simulink model "verify_House_OneNodeModel_mdl"  (R2016b)
settings: Solver=ode45  StartTime=0.0  StopTime=2*24*3600  MaxStep=100  RelTol=1e-3  EnableMultiTasking=on
libraries: carnot x5
settings Model: Creator=drhf  LastModifiedBy=drhf
settings DataIOCC: SaveFormat=Array  SignalLoggingSaveFormat=ModelDataLogs
settings OptimizationCC: ExpressionDepthLimit=2147483647  LifeSpan=inf
settings DebuggingCC: UnderspecifiedInitializationDetection=Classic  MergeDetectMultiDrivingBlocksExec=none  SolverPrmCheckMsg=warning  FcnCallInpInsideContextMsg=warning  StateNameClashWarn=warning  SFUnexpectedBacktrackingDiag=warning  SFNoUnconditionalDefaultTransitionDiag=warning  SFExecutionAtInitializationDiag=none
settings HardwareCC: ProdBitPerPointer=32  ProdBitPerSizeT=32  ProdBitPerPtrDiffT=32  ProdLargestAtomicFloat=None  ProdIntDivRoundTo=Undefined  ProdEndianess=Unspecified  ProdWordSize=32  ProdHWDeviceType=32-bit Generic
settings ModelReferenceCC: PropagateSignalLabelsOutOfModel=off
settings GRTTargetCC: TargetLangStandard=C89/C90 (ANSI)  GeneratePreprocessorConditionals=Disable all  CombineOutputUpdateFcns=off  GRTInterface=on
settings ConfigComp: CovMetricSettings=dw  CovHtmlReporting=on  CovSaveCumulativeToWorkspaceVar=on  CovSaveSingleToWorkspaceVar=on  CovExternalEMLEnable=off

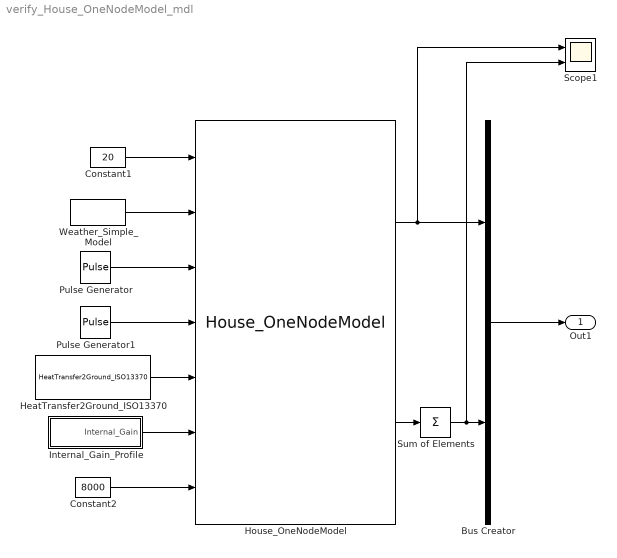
== system verify_House_OneNodeModel_mdl ==
  Bus Creator : BusCreator  Inputs=2
  Constant1 : Constant  Value=20
  Constant2 : Constant  Value=8000
  HeatTransfer2Ground_ISO13370 : carnot/Basic/Heat_Transfer/HeatTransfer2Ground_ISO13370  slabwidth=10  slablength=7  gammat=0  Tmeaninside=23.8  deltathetai=3.8  Tmeanoutside=11  deltathetae=9.3  tshift=319*3600  dwall=0.4  cond_ground=2.0  cp_ground=800  rho_ground=2500  utot=0.183
  House_OneNodeModel : carnot/Basic/Thermal_Models/House_OneNodeModel  A=140  UAout=0.197*(54.6+26.4)+0.286*((45.7+56.0)*2 -(12+4+3+4))  UAin=0  capa=0.5e6  tini=20  dtroom=inf  AziWin=[0 90 -180 -90]  Awin=[12 4 3 4]  Uwin="[1    1   1    1]*1.5"  Gwin="[1    1   1    1]*0.622*(1-0.15)"
  Internal_Gain_Profile : Subsystem
  Pulse Generator : DiscretePulseGenerator  PulseType=Time based  Period=24*3600  PulseWidth=50  PhaseDelay=12*3600
  Pulse Generator1 : DiscretePulseGenerator  PulseType=Time based  Amplitude=-1000  Period=24*3600  PulseWidth=50  PhaseDelay=12*3600
  Scope1 : Scope  NumInputPorts=2
  Sum of Elements : Sum  Inputs=+
  Weather_Simple_Model : carnot/Weather/Weather_Simple_Model  lat=60  Ibn=900  Idg=100  tamb=5  deltaTsky=-6  rh=50  precip="10e-3/24/3600           % 10 mm in 24 h"  cloud=0.125  p=1013e2  vw=1  wdir=270
  Out1 : Outport
  wires:
  House_OneNodeModel/1 -> Scope1/1, Bus Creator/1
  Bus Creator/1 -> Out1/1
  House_OneNodeModel/2 -> Sum of Elements/1
  Sum of Elements/1 -> Scope1/2, Bus Creator/2
  Pulse Generator/1 -> House_OneNodeModel/3
  Constant2/1 -> House_OneNodeModel/7
  Weather_Simple_Model/1 -> House_OneNodeModel/2
  Constant1/1 -> House_OneNodeModel/1
  Internal_Gain_Profile/1(Internal_Gain) -> House_OneNodeModel/6
  HeatTransfer2Ground_ISO13370/1 -> House_OneNodeModel/5
  Pulse Generator1/1 -> House_OneNodeModel/4

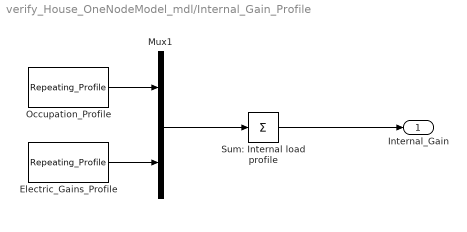
== system verify_House_OneNodeModel_mdl/Internal_Gain_Profile ==
  Electric_Gains_Profile : carnot/Load/General/Repeating_Profile  period=24*3600  rep_seq_t=[0 1 6 7 8 9 11 12 13 18 19 20 22 23]*3600  rep_seq_d=[1 5 1 1 1 2 1 1 4 2 1 2 1 1]*3600  rep_seq_y=[105 55 392.5 457.5 420 55 250 55 120 170 615 420 442.5 355]
  Mux1 : Mux  Inputs=2
  Occupation_Profile : carnot/Load/General/Repeating_Profile  period=24*3600  rep_seq_t=[0 6 7 8 9 11 12 13 14 15 17 18 20 21 22]*3600  rep_seq_d=[6 1 1 1 2 1 1 1 1 2 1 2 1 1 2]*3600  rep_seq_y=[4 2 3 2 0 1 3 2 1 0 1 2 4 3 4]*60
  Sum: Internal load profile : Sum  Inputs=+
  Internal_Gain : Outport
  wires:
  Sum: Internal load profile/1 -> Internal_Gain/1
  Electric_Gains_Profile/1 -> Mux1/2
  Occupation_Profile/1 -> Mux1/1
  Mux1/1 -> Sum: Internal load profile/1
